simulink model "RequirementTable_testing_RA"  (R2022b)
settings: Solver=FixedStepAuto  StartTime=0.0  StopTime=10.0  FixedStep=1e-3  RelTol=1e-3  EnableMultiTasking=on
undefined symbols (not defined in the file): D0, D1, D10, D11, D12, D13, D2, D3, D4, D5, D6, D7, D8, D9, PTA0, PTA1, PTA2, PTB23, PTB9, PTC16, PTC17, PTC2, PTC3, PTC4, PTD0, PTD1, PTD2, PTD3
libraries: frdmk64flib x18, dspstat3 x1
settings Model: SimulationMode=external  ExtModeTrigDuration=5  Creator=sarahalabdulrazzak  LastModifiedBy=TheCoaler
settings SolverCC: AlgebraicLoopSolver=TrustRegion
settings OptimizationCC: EnhancedBackFolding=on  PassReuseOutputArgsAs=Individual arguments  ZeroExternalMemoryAtStartup=off  ZeroInternalMemoryAtStartup=off  MaxStackSize=64  OptimizeBlockOrder=speed  DifferentSizesBufferReuse=on  OptimizationCustomize=off  EfficientTunableParamExpr=on
settings DebuggingCC: ParameterTunabilityLossMsg=error  UnconnectedInputMsg=warning  UnconnectedOutputMsg=warning  UnconnectedLineMsg=warning  SFMachineParentedDataDiag=warning
settings HardwareCC: ProdBitPerPointer=32  ProdBitPerSizeT=32  ProdBitPerPtrDiffT=32  ProdLargestAtomicInteger=Long  ProdLargestAtomicFloat=Double  ProdWordSize=32  ProdHWDeviceType=ARM Compatible->ARM Cortex
settings ModelReferenceCC: EnableRefExpFcnMdlSchedulingChecks=on
settings SFSimCC: MATLABDynamicMemAlloc=off
settings RTWCC: Description=Embedded Coder  SystemTargetFile=ert.tlc  HardwareBoard=NXP FRDM-K64F  TLCOptions="-aInlineSetEventsForThisBaseRateFcn=TLC_FALSE -aSuppressMultiTaskScheduler=TLC_FALSE  -aRateBasedStepFcn=0"  TemplateMakefile=ert_default_tmf  Toolchain=GNU Tools for ARM Embedded Processors
settings CodeAppCC: ForceParamTrailComments=on  IgnoreCustomStorageClasses=off  OperatorAnnotations=on  SimulinkDataObjDesc=on  SFDataObjDesc=on  InsertBlockDesc=on
settings ERTTargetCC: ExtMode=on  ExtModeTransport=4  ExtModeMexFile=sendToCommService  ExtModeMexArgs='RA_Modes' 0

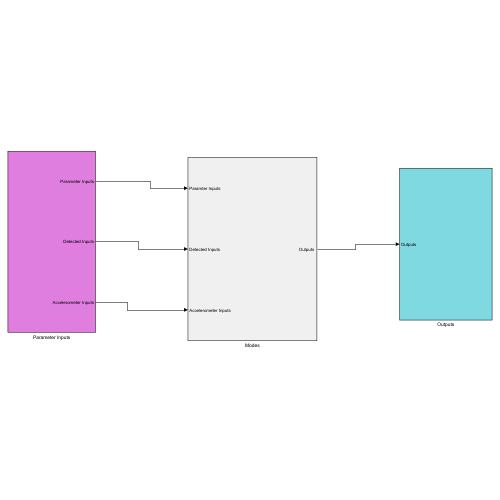
[thumbnail: Simulink's stored preview of the top-level diagram]
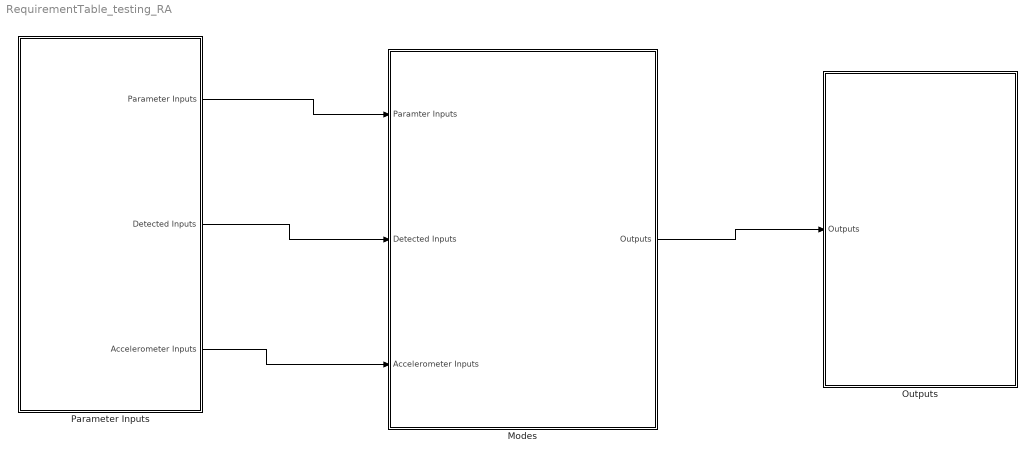
== system RequirementTable_testing_RA ==
  Modes : Subsystem
  Outputs : Subsystem
  Parameter Inputs : Subsystem
  wires:
  Parameter Inputs/1(Parameter Inputs) -> Modes/1(Paramter Inputs)
  Parameter Inputs/2(Detected Inputs) -> Modes/2(Detected Inputs)
  Modes/1("Outputs ") -> Outputs/1("Outputs ")
  Parameter Inputs/3(Accelerometer Inputs) -> Modes/3(Accelerometer Inputs)

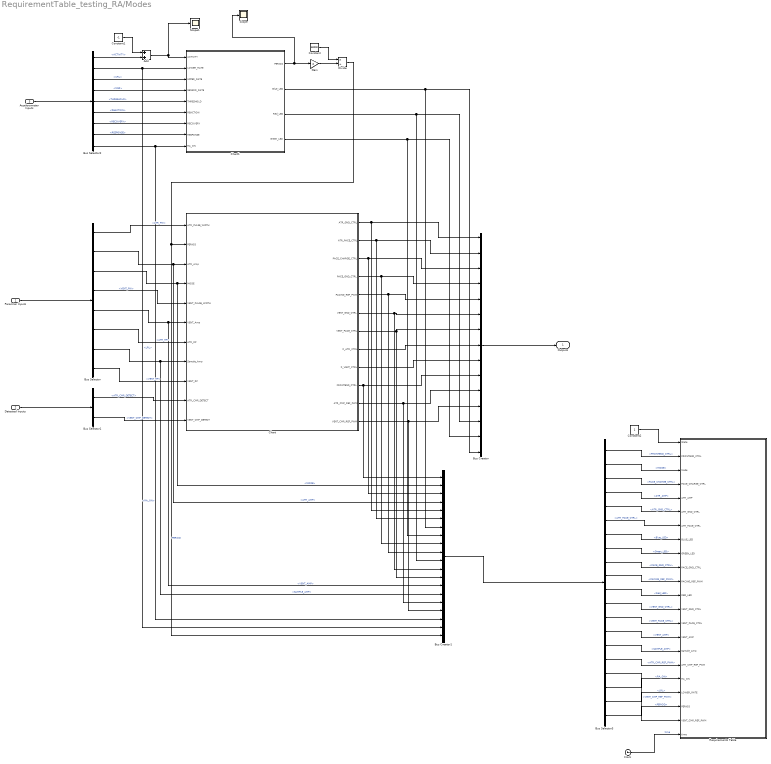
== system RequirementTable_testing_RA/Modes ==
  Paramter Inputs : Inport
  Detected Inputs : Inport  Port=2
  Accelerometer Inputs : Inport  Port=3
  Add : Sum
  Bus Creator : BusCreator  Inputs=15
  Bus Creator1 : BusCreator  Inputs=20
  Bus Selector : BusSelector  OutputSignals=ATR_PW,ATR_AMP,MODE,VENT_PW,VENT_AMP,ATR_RP,SAMPLE_AMP,VENT_RP
  Bus Selector1 : BusSelector  OutputSignals=ATR_CMP_DETECT,VENT_CMP_DETECT
  Bus Selector2 : BusSelector  OutputSignals=ACTIVITY,LRL,URL,MSR,THRESHOLD,REACTION,RECOVERY,RESPONSE,RA_ON
  Bus Selector3 : BusSelector  OutputSignals=FRONTEND_CTRL,MODE,PACE_CHARGE_CTRL,ATR_AMP,ATR_GND_CTRL,ATR_PACE_CTRL,Blue_LED,Green_LED,PACE_GND_CTRL,PACING_REF_PWM,Red_LED,VENT_GND_CTRL,VENT_PACE_CTRL,VENT_AMP,SAMPLE_AMP,ATR_CMP_REF_PWM,VENT_CMP_REF_PWM,RA_ON,LRL,PERIOD
  Chart : Stateflow chart  TreatAsAtomicUnit=on
  Chart1 : Stateflow chart  TreatAsAtomicUnit=on
  Clock : Clock
  Constant : Constant  Value=60000
  Constant1 : Constant  Value=-1
  Constant2 : Constant
  Divide : Product  Inputs=*/
  Gain : Gain  Gain=2
  Requirements Table : Requirements Table  TreatAsAtomicUnit=on
  Scope : Scope
  Scope1 : Scope
  "Outputs " : Outport
  wires:
  Paramter Inputs/1 -> Bus Selector/1
  Detected Inputs/1 -> Bus Selector1/1
  Bus Selector/1 -> Chart/1(ATR_PULSE_WIDTH)  "<ATR_PW>"
  Chart/1(ATR_GND_CTRL) -> Bus Creator1/5, Bus Creator/1
  Chart/2(ATR_PACE_CTRL) -> Bus Creator1/6, Bus Creator/2
  Chart/4(PACE_GND_CTRL) -> Bus Creator1/9, Bus Creator/4
  Chart/5(PACING_REF_PWM) -> Bus Creator1/10, Bus Creator/5
  Chart/6(VENT_GND_CTRL) -> Bus Creator1/12, Bus Creator/6
  Chart/7(VENT_PACE_CTRL) -> Bus Creator1/13, Bus Creator/7
  Chart/8(Z_ATR_CTRL) -> Bus Creator/8
  Chart/9(Z_VENT_CTRL) -> Bus Creator/9
  Chart/10(FRONTEND_CTRL) -> Bus Creator1/1, Bus Creator/10
  Chart/11(ATR_CMP_REF_PWM) -> Bus Creator1/16, Bus Creator/11
  Chart/12(VENT_CMP_REF_PWM) -> Bus Creator1/17, Bus Creator/12
  Bus Creator/1 -> "Outputs "/1
  Bus Selector1/1 -> Chart/10(ATR_CMP_DETECT)  "<ATR_CMP_DETECT>"
  Bus Selector1/2 -> Chart/11(VENT_CMP_DETECT)  "<VENT_CMP_DETECT>"
  Chart/3(PACE_CHARGE_CTRL) -> Bus Creator1/3, Bus Creator/3
  Bus Selector/2 -> Bus Creator1/4, Chart/3(ATR_Amp)  "<ATR_AMP>"
  Bus Selector/3 -> Bus Creator1/2, Chart/4(MODE)  "<MODE>"
  Bus Selector/4 -> Chart/5(VENT_PULSE_WIDTH)  "<VENT_PW>"
  Bus Selector/5 -> Bus Creator1/14, Chart/6(VENT_Amp)  "<VENT_AMP>"
  Bus Selector/6 -> Chart/7(ATR_RP)  "<ATR_RP>"
  Bus Selector/7 -> Bus Creator1/15, Chart/8(Sample_Amp)  "<SAMPLE_AMP>"
  Bus Selector/8 -> Chart/9(VENT_RP)  "<VENT_RP>"
  Accelerometer Inputs/1 -> Bus Selector2/1
  Bus Selector2/2 -> Bus Creator1/19, Chart1/2(LOWER_RATE)  "<LRL>"
  Bus Selector2/3 -> Chart1/3(UPPER_RATE)  "<URL>"
  Bus Selector2/4 -> Chart1/4(SENSOR_RATE)  "<MSR>"
  Bus Selector2/7 -> Chart1/7(RECOVERY)  "<RECOVERY>"
  Bus Selector2/8 -> Chart1/8(RESPONSE)  "<RESPONSE>"
  Bus Selector2/9 -> Bus Creator1/18, Chart1/9(RA_ON)  "<RA_ON>"
  Chart1/1(PERIOD) -> Scope/1, Gain/1
  Chart1/2(Blue_LED) -> Bus Creator1/7, Bus Creator/15
  Chart1/3(Red_LED) -> Bus Creator1/11, Bus Creator/13
  Chart1/4(Green_LED) -> Bus Creator1/8, Bus Creator/14
  Constant/1 -> Divide/1
  Divide/1 -> Bus Creator1/20, Chart/2(PERIOD)  "PERIOD"
  Gain/1 -> Divide/2
  Bus Selector2/5 -> Chart1/5(THRESHOLD)  "<THRESHOLD>"
  Bus Selector2/6 -> Chart1/6(REACTION)  "<REACTION>"
  Bus Selector2/1 -> Add/2  "<ACTIVITY>"
  Add/1 -> Scope1/1, Chart1/1(ACTIVITY)
  Constant1/1 -> Add/1
  Bus Creator1/1 -> Bus Selector3/1
  Bus Selector3/1 -> Requirements Table/2(FRONTEND_CTRL)  "<FRONTEND_CTRL>"
  Bus Selector3/2 -> Requirements Table/3(Mode)  "<MODE>"
  Bus Selector3/3 -> Requirements Table/4(PACE_CHARGE_CTRL)  "<PACE_CHARGE_CTRL>"
  Bus Selector3/4 -> Requirements Table/5(ATR_AMP)  "<ATR_AMP>"
  Bus Selector3/5 -> Requirements Table/6(ATR_GND_CTRL)  "<ATR_GND_CTRL>"
  Bus Selector3/6 -> Requirements Table/7(ATR_PACE_CTRL)  "<ATR_PACE_CTRL>"
  Bus Selector3/7 -> Requirements Table/8(BLUE_LED)  "<Blue_LED>"
  Bus Selector3/8 -> Requirements Table/9(GREEN_LED)  "<Green_LED>"
  Bus Selector3/9 -> Requirements Table/10(PACE_GND_CTRL)  "<PACE_GND_CTRL>"
  Bus Selector3/10 -> Requirements Table/11(PACING_REF_PWM)  "<PACING_REF_PWM>"
  Bus Selector3/11 -> Requirements Table/12(RED_LED)  "<Red_LED>"
  Bus Selector3/12 -> Requirements Table/13(VENT_GND_CTRL)  "<VENT_GND_CTRL>"
  Bus Selector3/13 -> Requirements Table/14(VENT_PACE_CTRL)  "<VENT_PACE_CTRL>"
  Bus Selector3/14 -> Requirements Table/15(VENT_AMP)  "<VENT_AMP>"
  Bus Selector3/15 -> Requirements Table/16(Sample_Amp)  "<SAMPLE_AMP>"
  Bus Selector3/16 -> Requirements Table/17(ATR_CMP_REF_PWM)  "<ATR_CMP_REF_PWM>"
  Bus Selector3/19 -> Requirements Table/19(LOWER_RATE)  "<LRL>"
  Constant2/1 -> Requirements Table/1(State)
  Bus Selector3/20 -> Requirements Table/20(PERIOD)  "<PERIOD>"
  Bus Selector3/18 -> Requirements Table/18(RA_ON)  "<RA_ON>"
  Bus Selector3/17 -> Requirements Table/21(VENT_CMP_REF_PWM)  "<VENT_CMP_REF_PWM>"
  Clock/1 -> Requirements Table/22(time)  "time"

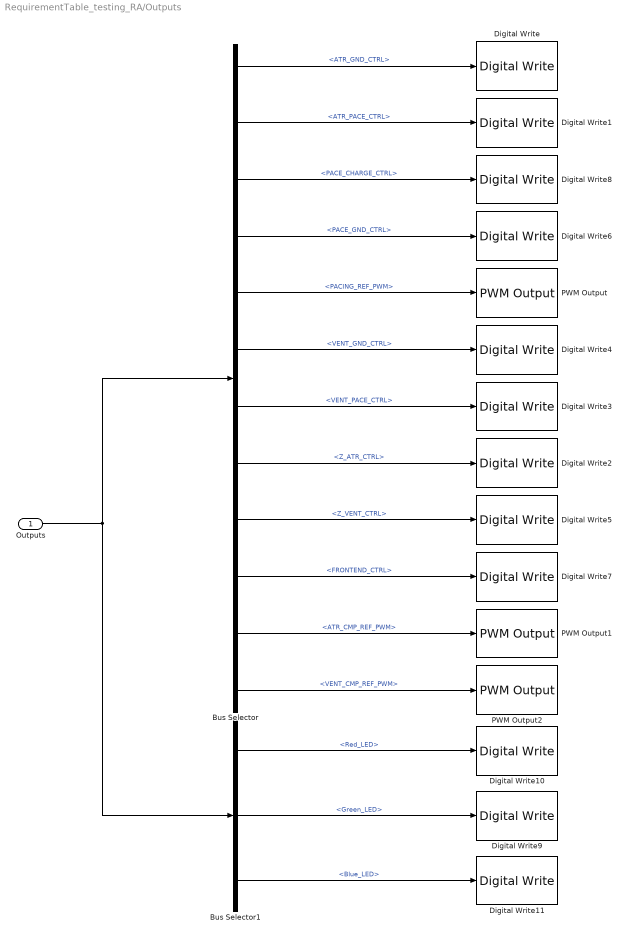
== system RequirementTable_testing_RA/Outputs ==
  "Outputs " : Inport
  Bus Selector : BusSelector  OutputSignals=ATR_GND_CTRL,ATR_PACE_CTRL,PACE_CHARGE_CTRL,PACE_GND_CTRL,PACING_REF_PWM,VENT_GND_CTRL,VENT_PACE_CTRL,Z_ATR_CTRL,Z_VENT_CTRL,FRONTEND_CTRL,ATR_CMP_REF_PWM,VENT_CMP_REF_PWM
  Bus Selector1 : BusSelector  OutputSignals=Red_LED,Green_LED,Blue_LED
  Digital Write : frdmk64flib/Digital Write  Whichpin=PTD2 (D11)
  Digital Write1 : frdmk64flib/Digital Write  Whichpin=PTA0 (D8)
  Digital Write10 : frdmk64flib/Digital Write  Whichpin=RED_LED
  Digital Write11 : frdmk64flib/Digital Write  Whichpin=BLUE_LED
  Digital Write2 : frdmk64flib/Digital Write  Whichpin=PTB23 (D4)
  Digital Write3 : frdmk64flib/Digital Write  Whichpin=PTC4 (D9)
  Digital Write4 : frdmk64flib/Digital Write  Whichpin=PTD3 (D12)
  Digital Write5 : frdmk64flib/Digital Write  Whichpin=PTC3 (D7)
  Digital Write6 : frdmk64flib/Digital Write  Whichpin=PTD0 (D10)
  Digital Write7 : frdmk64flib/Digital Write  Whichpin=PTD1 (D13)
  Digital Write8 : frdmk64flib/Digital Write  Whichpin=PTB9 (D2)
  Digital Write9 : frdmk64flib/Digital Write  Whichpin=GREEN_LED
  PWM Output : frdmk64flib/PWM Output  Whichpin=PTA2 (D5)  InitialFrequency=2000  InitialDutyCycle=0
  PWM Output1 : frdmk64flib/PWM Output  Whichpin=PTC2 (D6)  InitialFrequency=2000  InitialDutyCycle=0
  PWM Output2 : frdmk64flib/PWM Output  Whichpin=PTA1 (D3)  InitialFrequency=2000  InitialDutyCycle=0
  wires:
  Bus Selector/1 -> Digital Write/1  "<ATR_GND_CTRL>"
  Bus Selector/2 -> Digital Write1/1  "<ATR_PACE_CTRL>"
  Bus Selector/3 -> Digital Write8/1  "<PACE_CHARGE_CTRL>"
  Bus Selector/4 -> Digital Write6/1  "<PACE_GND_CTRL>"
  Bus Selector/5 -> PWM Output/1  "<PACING_REF_PWM>"
  Bus Selector/6 -> Digital Write4/1  "<VENT_GND_CTRL>"
  Bus Selector/7 -> Digital Write3/1  "<VENT_PACE_CTRL>"
  Bus Selector/8 -> Digital Write2/1  "<Z_ATR_CTRL>"
  Bus Selector/9 -> Digital Write5/1  "<Z_VENT_CTRL>"
  Bus Selector/10 -> Digital Write7/1  "<FRONTEND_CTRL>"
  Bus Selector/11 -> PWM Output1/1  "<ATR_CMP_REF_PWM>"
  Bus Selector/12 -> PWM Output2/1  "<VENT_CMP_REF_PWM>"
  "Outputs "/1 -> Bus Selector/1, Bus Selector1/1
  Bus Selector1/1 -> Digital Write10/1  "<Red_LED>"
  Bus Selector1/2 -> Digital Write9/1  "<Green_LED>"
  Bus Selector1/3 -> Digital Write11/1  "<Blue_LED>"

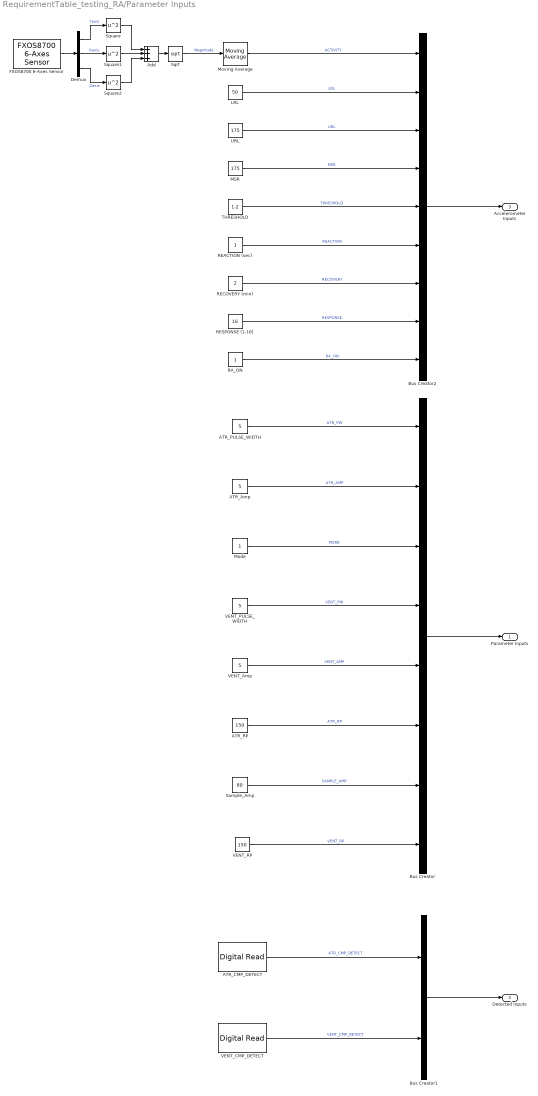
== system RequirementTable_testing_RA/Parameter Inputs ==
  ATR_Amp : Constant  Value=5
  ATR_CMP_DETECT : frdmk64flib/Digital Read  Whichpin=PTC16 (D0)  SampleTime=-1
  ATR_PULSE_WIDTH : Constant  Value=5
  ATR_RP : Constant  Value=150
  Add : Sum  Inputs=+++
  Bus Creator : BusCreator  Inputs=8
  Bus Creator1 : BusCreator  Inputs=2
  Bus Creator2 : BusCreator  Inputs=9
  Demux : Demux  Outputs=3
  FXOS8700 6-Axes Sensor : frdmk64flib/FXOS8700 6-Axes Sensor  Activesensor=Accelerometer only  ODR=800Hz  HybridODR=400Hz  Accelfullrange=-4g to +4g  SampleTime=-1
  LRL : Constant  Value=50  OutDataTypeStr=double
  MSR : Constant  Value=175  OutDataTypeStr=double
  Mode : Constant
  Moving Average : dspstat3/Moving Average  Method=Exponential weighting  ForgettingFactorPort=off  SpecifyWindowLength=on  WindowLength=4  OverlapLength=3  AllowArbitraryInputLength=off  ForgettingFactor=0.999  SimulateUsing=Code generation
  RA_ON : Constant  OutDataTypeStr=boolean
  REACTION (sec) : Constant  OutDataTypeStr=double
  RECOVERY (min) : Constant  Value=2  OutDataTypeStr=double
  RESPONSE (1-16) : Constant  Value=16  OutDataTypeStr=double
  Sample_Amp : Constant  Value=80
  Sqrt : Sqrt
  Square : Math  Operator=square
  Square1 : Math  Operator=square
  Square2 : Math  Operator=square
  THRESHOLD : Constant  Value=1.2  OutDataTypeStr=double
  URL : Constant  Value=175  OutDataTypeStr=double
  VENT_Amp : Constant  Value=5
  VENT_CMP_DETECT : frdmk64flib/Digital Read  Whichpin=PTC17 (D1)  SampleTime=-1
  VENT_PULSE_WIDTH : Constant  Value=5
  VENT_RP : Constant  Value=150
  Parameter Inputs : Outport
  Detected Inputs : Outport  Port=2
  Accelerometer Inputs : Outport  Port=3
  wires:
  Bus Creator/1 -> Parameter Inputs/1
  ATR_PULSE_WIDTH/1 -> Bus Creator/1  "ATR_PW"
  ATR_Amp/1 -> Bus Creator/2  "ATR_AMP"
  Mode/1 -> Bus Creator/3  "MODE"
  VENT_PULSE_WIDTH/1 -> Bus Creator/4  "VENT_PW"
  VENT_Amp/1 -> Bus Creator/5  "VENT_AMP"
  ATR_RP/1 -> Bus Creator/6  "ATR_RP"
  Sample_Amp/1 -> Bus Creator/7  "SAMPLE_AMP"
  VENT_RP/1 -> Bus Creator/8  "VENT_RP"
  Bus Creator1/1 -> Detected Inputs/1
  VENT_CMP_DETECT/1 -> Bus Creator1/2  "VENT_CMP_DETECT"
  ATR_CMP_DETECT/1 -> Bus Creator1/1  "ATR_CMP_DETECT"
  Sqrt/1 -> Moving Average/1  "Magnitude"
  Demux/3 -> Square2/1  "Zaxis"
  Square2/1 -> Add/3
  Add/1 -> Sqrt/1
  Demux/2 -> Square1/1  "Xaxis"
  Square/1 -> Add/1
  Demux/1 -> Square/1  "Yaxis"
  FXOS8700 6-Axes Sensor/1 -> Demux/1
  Square1/1 -> Add/2
  Bus Creator2/1 -> Accelerometer Inputs/1
  Moving Average/1 -> Bus Creator2/1  "ACTIVITY"
  LRL/1 -> Bus Creator2/2  "LRL"
  URL/1 -> Bus Creator2/3  "URL"
  MSR/1 -> Bus Creator2/4  "MSR"
  RA_ON/1 -> Bus Creator2/9  "RA_ON"
  REACTION (sec)/1 -> Bus Creator2/6  "REACTION"
  THRESHOLD/1 -> Bus Creator2/5  "THRESHOLD"
  RECOVERY (min)/1 -> Bus Creator2/7  "RECOVERY"
  RESPONSE (1-16)/1 -> Bus Creator2/8  "RESPONSE"

== stateflow chart RequirementTable_testing_RA/Modes/Chart1 ==
  state RECOVER_RATE
    %this is for if the RA is turned off while the
    %slowly shift activity (might not need)
    %if the period is above LRL, reduce by amount that will bring diff to 0 within recovery time
    Green_LED = true
    AVG_ACT = ACTIVITY
    if PERIOD > LOWER_RATE
    PERIOD = PERIOD - (SENSOR_RATE-LOWER_RATE)/(RECOVERY*1000)
    DELAY = (RECOVERY*1000)
    else
    PERIOD = LOWER_RATE
    DELAY = 0
    end
  state RA_OFF
    %set the period to LRL
    %read current activity
    %and assign to var.
    entry:
    PERIOD = LOWER_RATE
    AVG_ACT = ACTIVITY
    TH = single(THRESHOLD)
  state SET_TARGET
    %set the target rate and make sure it falls within the bounds
    Green_LED = false
    Red_LED = true
    TARGET_RATE = RESPONSE*((SENSOR_RATE - LOWER_RATE)/10)*ACTIVITY + LOWER_RATE
    %TARGET_RATE = 120
    if TARGET_RATE > SENSOR_RATE
    TARGET_RATE = SENSOR_RATE
    elseif TARGET_RATE < LOWER_RATE
    TARGET_RATE = LOWER_RATE
    end
  state RA_ON
    entry:
    Blue_LED = false
    Green_LED = false
    %Red_LED = false
  state RECOVER_REACT
    %slowly shift activity (might not need)
    %if Period is above target, decrease using recovery
    %if below target, increase using reaction
    Blue_LED = true
    AVG_ACT = ACTIVITY
    if PERIOD > TARGET_RATE
    PERIOD = PERIOD - (SENSOR_RATE-LOWER_RATE)/(RECOVERY*1000)
    DELAY = (RECOVERY*1000)
    elseif PERIOD < TARGET_RATE
    PERIOD = PERIOD + (SENSOR_RATE-LOWER_RATE)/(REACTION*1000)
    DELAY = (REACTION*1000)
    end
  RECOVER_RATE -> SET_TARGET [order 1] : [n >= DELAY && AVG_ACT >= TH]
  RECOVER_RATE -> RECOVER_RATE [order 2] : after(1,msec){n = n+1}
  RECOVER_RATE -> RA_OFF [order 3] : [RA_ON == FALSE && n >= DELAY]
  RA_ON -> RECOVER_RATE [order 1] : [AVG_ACT < TH]{n=0}
  (default) -> RA_OFF
  RA_ON -> SET_TARGET [order 2] : [AVG_ACT >= TH]
  RA_OFF -> RA_ON : [RA_ON == TRUE]{TARGET_RATE=PERIOD}
  RECOVER_REACT -> RA_ON [order 1] : [n >= DELAY]
  SET_TARGET -> RECOVER_REACT : {n=0, AVG_ACT = ACTIVITY}
  RECOVER_REACT -> RECOVER_REACT [order 2] : after(1,msec){n = n+1}
  data: ACTIVITY input; LOWER_RATE input; UPPER_RATE input; SENSOR_RATE input; THRESHOLD input; REACTION input; RECOVERY input; RESPONSE input; RA_ON input; PERIOD output double; TRUE local =1; FALSE local =0; TARGET_RATE local double; DELAY local double; n local; Blue_LED output; Red_LED output; Green_LED output; TH local; AVG_ACT local

== stateflow chart RequirementTable_testing_RA/Modes/Requirements Table ==
  (default) -> (junction 1073748085)
  (junction 1073748085) -> (junction 1073748086) : {
      | % SF_REQ_REV_07
      | }
  (junction 1073748086) -> (junction 1073748088) : {
      | % HEADER_ASSIGNMENTS
      |
      | }
  (junction 1073748088) -> (junction 1073748418) : {
      | % START_A_28
      | }
  (junction 1073748418) -> (junction 1073748420) : {
      | }
  (junction 1073748420) -> (junction 1073748422) : {
      | reqtable_assumption((Mode<=4), 28);
      | }
  (junction 1073748422) -> (junction 1073748424) : {
      | }
  (junction 1073748424) -> (junction 1073748426) : {
      | % START_A_109
      | }
  (junction 1073748426) -> (junction 1073748428) : {
      | }
  (junction 1073748428) -> (junction 1073748430) : {
      | reqtable_assumption((Mode>=1), 109);
      | }
  (junction 1073748430) -> (junction 1073748432) : {
      | }
  (junction 1073748432) -> (junction 1073748434) : {
      | % END_A_109
      | }
  (junction 1073748434) -> (junction 1073748440) : {
      | % START_A_112
      | }
  (junction 1073748440) -> (junction 1073748442) : {
      | }
  (junction 1073748442) -> (junction 1073748444) : {
      | reqtable_assumption((rem(Mode,1)<=0), 112);
      | }
  (junction 1073748444) -> (junction 1073748446) : {
      | }
  (junction 1073748446) -> (junction 1073748448) : {
      | % END_A_112
      | }
  (junction 1073748448) -> (junction 1073748436) : {
      | % END_A_28
      | }
  (junction 1073748436) -> (junction 1073748464) : {
      | % START_A_106
      | }
  (junction 1073748464) -> (junction 1073748466) : {
      | }
  (junction 1073748466) -> (junction 1073748468) : {
      | reqtable_assumption((State<=1), 106);
      | }
  (junction 1073748468) -> (junction 1073748470) : {
      | }
  (junction 1073748470) -> (junction 1073748472) : {
      | % START_A_118
      | }
  (junction 1073748472) -> (junction 1073748474) : {
      | }
  (junction 1073748474) -> (junction 1073748476) : {
      | reqtable_assumption((State>=0), 118);
      | }
  (junction 1073748476) -> (junction 1073748478) : {
      | }
  (junction 1073748478) -> (junction 1073748480) : {
      | % END_A_118
      | }
  (junction 1073748480) -> (junction 1073748482) : {
      | % END_A_106
      | }
  (junction 1073748482) -> (junction 1073748486) : {
      | % START_A_115
      | }
  (junction 1073748486) -> (junction 1073748488) : {
      | }
  (junction 1073748488) -> (junction 1073748490) : {
      | reqtable_assumption((FRONTEND_CTRL<=1), 115);
      | }
  (junction 1073748490) -> (junction 1073748492) : {
      | }
  (junction 1073748492) -> (junction 1073748494) : {
      | % START_A_121
      | }
  (junction 1073748494) -> (junction 1073748496) : {
      | }
  (junction 1073748496) -> (junction 1073748498) : {
      | reqtable_assumption((FRONTEND_CTRL>=0), 121);
      | }
  (junction 1073748498) -> (junction 1073748500) : {
      | }
  (junction 1073748500) -> (junction 1073748502) : {
      | % END_A_121
      | }
  (junction 1073748502) -> (junction 1073748504) : {
      | % END_A_115
      | }
  (junction 1073748504) -> (junction 1073748100) : {
      | % START_R_1
      | }
  (junction 1073748100) -> (junction 1073748102) : {
      | }
  (junction 1073748102) -> (junction 1073748104)
  (junction 1073748104) -> (junction 1073748106) [order 1] : [(((RA_ON) == (0))) && (((Mode) == (1))) && (((State) == (0)))]
  (junction 1073748104) -> (junction 1073748112) [order 2]
  (junction 1073748106) -> (junction 1073748108) : {
      | reqtable_postcondition((((PACE_CHARGE_CTRL) == (1))) && (ATR_PACE_CTRL == 0) && (((PACING_REF_PWM ) == (ATR_AMP))) && (((PACE_CHARGE_CTRL) == (1))) && (((PACE_GND_CTRL) == (1))) && (ATR_GND_CTRL == 1) && (((RED_LED) == (0))) && (((GREEN_LED) == (0))) && (((BLUE_LED) == (0))) && (time-oldTime / (60*1000) >= LOWER_RATE), 'R:1');
      |
      | }
  (junction 1073748108) -> (junction 1073748110) : {
      | }
  (junction 1073748110) -> (junction 1073748112)
  (junction 1073748112) -> (junction 1073748114)
  (junction 1073748114) -> (junction 1073748116) : {
      | % END_R_1
      | }
  (junction 1073748116) -> (junction 1073748118) : {
      | % START_R_82
      | }
  (junction 1073748118) -> (junction 1073748120) : {
      | }
  (junction 1073748120) -> (junction 1073748122)
  (junction 1073748122) -> (junction 1073748124) [order 1] : [(((RA_ON) == (1))) && (((Mode) == (1))) && (((State) == (0)))]
  (junction 1073748122) -> (junction 1073748130) [order 2]
  (junction 1073748124) -> (junction 1073748126) : {
      | reqtable_postcondition((((PACE_CHARGE_CTRL) == (1))) && (ATR_PACE_CTRL == 0) && (((PACING_REF_PWM ) == (ATR_AMP))) && (((PACE_CHARGE_CTRL) == (1))) && (((PACE_GND_CTRL) == (1))) && (ATR_GND_CTRL == 1) && (((RED_LED) == (0))) && (((GREEN_LED) == (0))) && (((BLUE_LED) == (0))) && (time-oldTime >= PERIOD-5), 'R:2');
      |
      | }
  (junction 1073748126) -> (junction 1073748128) : {
      | }
  (junction 1073748128) -> (junction 1073748130)
  (junction 1073748130) -> (junction 1073748132)
  (junction 1073748132) -> (junction 1073748134) : {
      | % END_R_82
      | }
  (junction 1073748134) -> (junction 1073748136) : {
      | % START_R_7
      | }
  (junction 1073748136) -> (junction 1073748138) : {
      | }
  (junction 1073748138) -> (junction 1073748140)
  (junction 1073748140) -> (junction 1073748142) [order 1] : [(((RA_ON) == (0))) && (((Mode) == (1))) && (((State) == (1)))]
  (junction 1073748140) -> (junction 1073748148) [order 2]
  (junction 1073748142) -> (junction 1073748144) : {
      | reqtable_postcondition((((PACE_CHARGE_CTRL) == (0))) && (ATR_PACE_CTRL == 1) && (((PACING_REF_PWM ) == (ATR_AMP))) && (((PACE_CHARGE_CTRL) == (0))) && (((PACE_GND_CTRL) == (1))) && (ATR_GND_CTRL == 0) && (((RED_LED) == (1))) && (((GREEN_LED) == (0))) && (((BLUE_LED) == (0))) && (time-oldTime / (60*1000) >= LOWER_RATE), 'R:3');
      |
      | }
  (junction 1073748144) -> (junction 1073748146) : {
      | }
  (junction 1073748146) -> (junction 1073748148)
  (junction 1073748148) -> (junction 1073748150)
  (junction 1073748150) -> (junction 1073748152) : {
      | % END_R_7
      | }
  (junction 1073748152) -> (junction 1073748154) : {
      | % START_R_88
      | }
  (junction 1073748154) -> (junction 1073748156) : {
      | }
  (junction 1073748156) -> (junction 1073748158)
  (junction 1073748158) -> (junction 1073748160) [order 1] : [(((RA_ON) == (1))) && (((Mode) == (1))) && (((State) == (1)))]
  (junction 1073748158) -> (junction 1073748166) [order 2]
  (junction 1073748160) -> (junction 1073748162) : {
      | reqtable_postcondition((((PACE_CHARGE_CTRL) == (0))) && (ATR_PACE_CTRL == 1) && (((PACING_REF_PWM ) == (ATR_AMP))) && (((PACE_CHARGE_CTRL) == (0))) && (((PACE_GND_CTRL) == (1))) && (ATR_GND_CTRL == 0) && (((RED_LED) == (1))) && (((GREEN_LED) == (0))) && (((BLUE_LED) == (0))) && (time-oldTime >= PERIOD-5), 'R:4');
      |
      | }
  (junction 1073748162) -> (junction 1073748164) : {
      | }
  (junction 1073748164) -> (junction 1073748166)
  (junction 1073748166) -> (junction 1073748168)
  (junction 1073748168) -> (junction 1073748170) : {
      | % END_R_88
      | }
  (junction 1073748170) -> (junction 1073748172) : {
      | % START_R_10
      | }
  (junction 1073748172) -> (junction 1073748174) : {
      | }
  (junction 1073748174) -> (junction 1073748176)
  (junction 1073748176) -> (junction 1073748178) [order 1] : [(((RA_ON) == (0))) && (((Mode) == (3))) && (((State) == (0)))]
  (junction 1073748176) -> (junction 1073748184) [order 2]
  (junction 1073748178) -> (junction 1073748180) : {
      | reqtable_postcondition((((PACE_CHARGE_CTRL) == (1))) && (VENT_PACE_CTRL == 0) && (((PACING_REF_PWM ) == (VENT_AMP))) && (((PACE_CHARGE_CTRL) == (1))) && (((PACE_GND_CTRL) == (1))) && (VENT_GND_CTRL == 1) && (((RED_LED) == (0))) && (((GREEN_LED) == (0))) && (((BLUE_LED) == (0))) && (time-oldTime / (60*1000) >= LOWER_RATE), 'R:5');
      |
      | }
  (junction 1073748180) -> (junction 1073748182) : {
      | }
  (junction 1073748182) -> (junction 1073748184)
  (junction 1073748184) -> (junction 1073748186)
  (junction 1073748186) -> (junction 1073748188) : {
      | % END_R_10
      | }
  (junction 1073748188) -> (junction 1073748190) : {
      | % START_R_85
      | }
  (junction 1073748190) -> (junction 1073748192) : {
      | }
  (junction 1073748192) -> (junction 1073748194)
  (junction 1073748194) -> (junction 1073748196) [order 1] : [(((RA_ON) == (1))) && (((Mode) == (3))) && (((State) == (0)))]
  (junction 1073748194) -> (junction 1073748202) [order 2]
  (junction 1073748196) -> (junction 1073748198) : {
      | reqtable_postcondition((((PACE_CHARGE_CTRL) == (1))) && (VENT_PACE_CTRL == 0) && (((PACING_REF_PWM ) == (VENT_AMP))) && (((PACE_CHARGE_CTRL) == (1))) && (((PACE_GND_CTRL) == (1))) && (VENT_GND_CTRL == 1) && (((RED_LED) == (0))) && (((GREEN_LED) == (0))) && (((BLUE_LED) == (0))) && (time-oldTime >= PERIOD-5), 'R:6');
      |
      | }
  (junction 1073748198) -> (junction 1073748200) : {
      | }
  (junction 1073748200) -> (junction 1073748202)
  (junction 1073748202) -> (junction 1073748204)
  (junction 1073748204) -> (junction 1073748206) : {
      | % END_R_85
      | }
  (junction 1073748206) -> (junction 1073748208) : {
      | % START_R_13
      | }
  (junction 1073748208) -> (junction 1073748210) : {
      | }
  (junction 1073748210) -> (junction 1073748212)
  (junction 1073748212) -> (junction 1073748214) [order 1] : [(((RA_ON) == (0))) && (((Mode) == (3))) && (((State) == (1)))]
  (junction 1073748212) -> (junction 1073748220) [order 2]
  (junction 1073748214) -> (junction 1073748216) : {
      | reqtable_postcondition((((PACE_CHARGE_CTRL) == (0))) && (VENT_PACE_CTRL == 1) && (((PACING_REF_PWM ) == (VENT_AMP))) && (((PACE_CHARGE_CTRL) == (0))) && (((PACE_GND_CTRL) == (1))) && (VENT_GND_CTRL == 0) && (((RED_LED) == (0))) && (((GREEN_LED) == (1))) && (((BLUE_LED) == (0))) && (time-oldTime / (60*1000) >= LOWER_RATE), 'R:7');
      |
      | }
  (junction 1073748216) -> (junction 1073748218) : {
      | }
  (junction 1073748218) -> (junction 1073748220)
  (junction 1073748220) -> (junction 1073748222)
  (junction 1073748222) -> (junction 1073748224) : {
      | % END_R_13
      | }
  (junction 1073748224) -> (junction 1073748226) : {
      | % START_R_91
      | }
  (junction 1073748226) -> (junction 1073748228) : {
      | }
  (junction 1073748228) -> (junction 1073748230)
  (junction 1073748230) -> (junction 1073748232) [order 1] : [(((RA_ON) == (1))) && (((Mode) == (3))) && (((State) == (1)))]
  (junction 1073748230) -> (junction 1073748238) [order 2]
  (junction 1073748232) -> (junction 1073748234) : {
      | reqtable_postcondition((((PACE_CHARGE_CTRL) == (0))) && (VENT_PACE_CTRL == 1) && (((PACING_REF_PWM ) == (VENT_AMP))) && (((PACE_CHARGE_CTRL) == (0))) && (((PACE_GND_CTRL) == (1))) && (VENT_GND_CTRL == 0) && (((RED_LED) == (0))) && (((GREEN_LED) == (1))) && (((BLUE_LED) == (0))) && (time-oldTime >= PERIOD-5), 'R:8');
      |
      | }
  (junction 1073748234) -> (junction 1073748236) : {
      | }
  (junction 1073748236) -> (junction 1073748238)
  (junction 1073748238) -> (junction 1073748240)
  (junction 1073748240) -> (junction 1073748242) : {
      | % END_R_91
      | }
  (junction 1073748242) -> (junction 1073748244) : {
      | % START_R_16
      | }
  (junction 1073748244) -> (junction 1073748246) : {
      | }
  (junction 1073748246) -> (junction 1073748248)
  (junction 1073748248) -> (junction 1073748250) [order 1] : [(((RA_ON) == (0))) && (((Mode) == (2))) && (((State) == (0))) && (FRONTEND_CTRL == 1)]
  (junction 1073748248) -> (junction 1073748256) [order 2]
  (junction 1073748250) -> (junction 1073748252) : {
      | reqtable_postcondition((((PACE_CHARGE_CTRL) == (1))) && (ATR_PACE_CTRL == 0) && (((PACING_REF_PWM ) == (ATR_AMP))) && (((PACE_CHARGE_CTRL) == (1))) && (((PACE_GND_CTRL) == (1))) && (ATR_GND_CTRL == 1) && (((RED_LED) == (0))) && (((GREEN_LED) == (0))) && (((BLUE_LED) == (0))) && (ATR_CMP_REF_PWM == Sample_Amp) && (time-oldTime / (60*1000) >= LOWER_RATE), 'R:9');
      |
      | }
  (junction 1073748252) -> (junction 1073748254) : {
      | }
  (junction 1073748254) -> (junction 1073748256)
  (junction 1073748256) -> (junction 1073748258)
  (junction 1073748258) -> (junction 1073748260) : {
      | % END_R_16
      | }
  (junction 1073748260) -> (junction 1073748262) : {
      | % START_R_94
      | }
  (junction 1073748262) -> (junction 1073748264) : {
      | }
  (junction 1073748264) -> (junction 1073748266)
  (junction 1073748266) -> (junction 1073748268) [order 1] : [(((RA_ON) == (1))) && (((Mode) == (2))) && (((State) == (0))) && (FRONTEND_CTRL == 1)]
  (junction 1073748266) -> (junction 1073748274) [order 2]
  (junction 1073748268) -> (junction 1073748270) : {
      | reqtable_postcondition((((PACE_CHARGE_CTRL) == (1))) && (ATR_PACE_CTRL == 0) && (((PACING_REF_PWM ) == (ATR_AMP))) && (((PACE_CHARGE_CTRL) == (1))) && (((PACE_GND_CTRL) == (1))) && (ATR_GND_CTRL == 1) && (((RED_LED) == (0))) && (((GREEN_LED) == (0))) && (((BLUE_LED) == (0))) && (ATR_CMP_REF_PWM == Sample_Amp) && (time-oldTime >= PERIOD-5), 'R:10');
      |
      | }
  (junction 1073748270) -> (junction 1073748272) : {
      | }
  (junction 1073748272) -> (junction 1073748274)
  (junction 1073748274) -> (junction 1073748276)
  (junction 1073748276) -> (junction 1073748278) : {
      | % END_R_94
      | }
  (junction 1073748278) -> (junction 1073748280) : {
      | % START_R_19
      | }
  (junction 1073748280) -> (junction 1073748282) : {
      | }
  (junction 1073748282) -> (junction 1073748284)
  (junction 1073748284) -> (junction 1073748286) [order 1] : [(((RA_ON) == (0))) && (((Mode) == (2))) && (((State) == (1)))]
  (junction 1073748284) -> (junction 1073748292) [order 2]
  (junction 1073748286) -> (junction 1073748288) : {
      | reqtable_postcondition((((PACE_CHARGE_CTRL) == (0))) && (ATR_PACE_CTRL == 1) && (((PACING_REF_PWM ) == (ATR_AMP))) && (((PACE_CHARGE_CTRL) == (0))) && (((PACE_GND_CTRL) == (1))) && (ATR_GND_CTRL == 0) && (((RED_LED) == (0))) && (((GREEN_LED) == (0))) && (((BLUE_LED) == (0))) && (ATR_CMP_REF_PWM == Sample_Amp) && (time-oldTime / (60*1000) >= LOWER_RATE), 'R:11');
      |
      | }
  (junction 1073748288) -> (junction 1073748290) : {
      | }
  (junction 1073748290) -> (junction 1073748292)
  (junction 1073748292) -> (junction 1073748294)
  (junction 1073748294) -> (junction 1073748296) : {
      | % END_R_19
      | }
  (junction 1073748296) -> (junction 1073748298) : {
      | % START_R_97
      | }
  (junction 1073748298) -> (junction 1073748300) : {
      | }
  (junction 1073748300) -> (junction 1073748302)
  (junction 1073748302) -> (junction 1073748304) [order 1] : [(((RA_ON) == (1))) && (((Mode) == (2))) && (((State) == (1)))]
  (junction 1073748302) -> (junction 1073748310) [order 2]
  (junction 1073748304) -> (junction 1073748306) : {
      | reqtable_postcondition((((PACE_CHARGE_CTRL) == (0))) && (ATR_PACE_CTRL == 1) && (((PACING_REF_PWM ) == (ATR_AMP))) && (((PACE_CHARGE_CTRL) == (0))) && (((PACE_GND_CTRL) == (1))) && (ATR_GND_CTRL == 0) && (((RED_LED) == (0))) && (((GREEN_LED) == (0))) && (((BLUE_LED) == (0))) && (ATR_CMP_REF_PWM == Sample_Amp) && (time-oldTime >= PERIOD-5), 'R:12');
      |
      | }
  (junction 1073748306) -> (junction 1073748308) : {
      | }
  (junction 1073748308) -> (junction 1073748310)
  (junction 1073748310) -> (junction 1073748312)
  (junction 1073748312) -> (junction 1073748314) : {
      | % END_R_97
      | }
  (junction 1073748314) -> (junction 1073748316) : {
      | % START_R_22
      | }
  (junction 1073748316) -> (junction 1073748318) : {
      | }
  (junction 1073748318) -> (junction 1073748320)
  (junction 1073748320) -> (junction 1073748322) [order 1] : [(((RA_ON) == (0))) && (((Mode) == (4))) && (((State) == (0))) && (FRONTEND_CTRL == 1)]
  (junction 1073748320) -> (junction 1073748328) [order 2]
  (junction 1073748322) -> (junction 1073748324) : {
      | reqtable_postcondition((((PACE_CHARGE_CTRL) == (1))) && (VENT_PACE_CTRL == 0) && (((PACING_REF_PWM ) == (VENT_AMP))) && (((PACE_CHARGE_CTRL) == (1))) && (((PACE_GND_CTRL) == (1))) && (VENT_GND_CTRL == 1) && (((RED_LED) == (0))) && (((GREEN_LED) == (0))) && (((BLUE_LED) == (0))) && (VENT_CMP_REF_PWM == Sample_Amp) && (time-oldTime / (60*1000) >= LOWER_RATE), 'R:13');
      |
      | }
  (junction 1073748324) -> (junction 1073748326) : {
      | }
  (junction 1073748326) -> (junction 1073748328)
  (junction 1073748328) -> (junction 1073748330)
  (junction 1073748330) -> (junction 1073748332) : {
      | % END_R_22
      | }
  (junction 1073748332) -> (junction 1073748334) : {
      | % START_R_100
      | }
  (junction 1073748334) -> (junction 1073748336) : {
      | }
  (junction 1073748336) -> (junction 1073748338)
  (junction 1073748338) -> (junction 1073748340) [order 1] : [(((RA_ON) == (1))) && (((Mode) == (4))) && (((State) == (0))) && (FRONTEND_CTRL == 1)]
  (junction 1073748338) -> (junction 1073748346) [order 2]
  (junction 1073748340) -> (junction 1073748342) : {
      | reqtable_postcondition((((PACE_CHARGE_CTRL) == (1))) && (VENT_PACE_CTRL == 0) && (((PACING_REF_PWM ) == (VENT_AMP))) && (((PACE_CHARGE_CTRL) == (1))) && (((PACE_GND_CTRL) == (1))) && (VENT_GND_CTRL == 1) && (((RED_LED) == (0))) && (((GREEN_LED) == (0))) && (((BLUE_LED) == (0))) && (VENT_CMP_REF_PWM == Sample_Amp) && (time-oldTime >= PERIOD-5), 'R:14');
      |
      | }
  (junction 1073748342) -> (junction 1073748344) : {
      | }
  (junction 1073748344) -> (junction 1073748346)
  (junction 1073748346) -> (junction 1073748348)
  (junction 1073748348) -> (junction 1073748350) : {
      | % END_R_100
      | }
  (junction 1073748350) -> (junction 1073748352) : {
      | % START_R_25
      | }
  (junction 1073748352) -> (junction 1073748354) : {
      | }
  (junction 1073748354) -> (junction 1073748356)
  (junction 1073748356) -> (junction 1073748358) [order 1] : [(((RA_ON) == (0))) && (((Mode) == (4))) && (((State) == (1)))]
  (junction 1073748356) -> (junction 1073748364) [order 2]
  (junction 1073748358) -> (junction 1073748360) : {
      | reqtable_postcondition((((PACE_CHARGE_CTRL) == (0))) && (VENT_PACE_CTRL == 1) && (((PACING_REF_PWM ) == (VENT_AMP))) && (((PACE_CHARGE_CTRL) == (0))) && (((PACE_GND_CTRL) == (1))) && (VENT_GND_CTRL == 0) && (((RED_LED) == (0))) && (((GREEN_LED) == (1))) && (((BLUE_LED) == (0))) && (VENT_CMP_REF_PWM == Sample_Amp) && (time-oldTime / (60*1000) >= LOWER_RATE), 'R:15');
      |
      | }
  (junction 1073748360) -> (junction 1073748362) : {
      | }
  (junction 1073748362) -> (junction 1073748364)
  (junction 1073748364) -> (junction 1073748366)
  (junction 1073748366) -> (junction 1073748368) : {
      | % END_R_25
      | }
  (junction 1073748368) -> (junction 1073748370) : {
      | % START_R_103
      | }
  (junction 1073748370) -> (junction 1073748372) : {
      | }
  (junction 1073748372) -> (junction 1073748374)
  (junction 1073748374) -> (junction 1073748376) [order 1] : [(((RA_ON) == (1))) && (((Mode) == (4))) && (((State) == (1)))]
  (junction 1073748374) -> (junction 1073748382) [order 2]
  (junction 1073748376) -> (junction 1073748378) : {
      | reqtable_postcondition((((PACE_CHARGE_CTRL) == (0))) && (VENT_PACE_CTRL == 1) && (((PACING_REF_PWM ) == (VENT_AMP))) && (((PACE_CHARGE_CTRL) == (0))) && (((PACE_GND_CTRL) == (1))) && (VENT_GND_CTRL == 0) && (((RED_LED) == (0))) && (((GREEN_LED) == (1))) && (((BLUE_LED) == (0))) && (VENT_CMP_REF_PWM == Sample_Amp) && (time-oldTime >= PERIOD-5), 'R:16');
      |
      | }
  (junction 1073748378) -> (junction 1073748380) : {
      | }
  (junction 1073748380) -> (junction 1073748382)
  (junction 1073748382) -> (junction 1073748384)
  (junction 1073748384) -> (junction 1073748386) : {
      | % END_R_103
      | }
  data: State input; FRONTEND_CTRL input; Mode input; PACE_CHARGE_CTRL input; ATR_AMP input; ATR_GND_CTRL input; ATR_PACE_CTRL input; BLUE_LED input; GREEN_LED input; PACE_GND_CTRL input; PACING_REF_PWM input; RED_LED input; VENT_GND_CTRL input; VENT_PACE_CTRL input; VENT_AMP input; Sample_Amp input; ATR_CMP_REF_PWM input; RA_ON input; LOWER_RATE input; PERIOD input; VENT_CMP_REF_PWM input; time input double [0..]; oldTime constant double =0

== stateflow chart RequirementTable_testing_RA/Modes/Chart ==
  state Identify_Mode_Path
    entry:
    % MODE = 1 (AOO)
    % MODE = 2 (AAI)
    % MODE = 3 (VOO)
    % MODE = 4 (VVI)
    %
    %pacemaker disconnected
    %stop sensing
    PACE_CHARGE_CTRL = LOW
    VENT_PACE_CTRL = LOW
    ATR_PACE_CTRL = LOW
    PACE_GND_CTRL = LOW
    ATR_GND_CTRL = LOW
    VENT_GND_CTRL = LOW
    Z_ATR_CTRL = LOW
    Z_VENT_CTRL = LOW
    FRONTEND_CTRL = LOW
  state AOO
    entry:
    %Charge primary capcitor C22
    ATR_PACE_CTRL=LOW
    PACING_REF_PWM = 20*ATR_Amp
    PACE_CHARGE_CTRL = HIGH
    %Discharge block capacitor C21
    PACE_GND_CTRL = HIGH
    ATR_GND_CTRL = HIGH
    %use LED  to verify state
  state AOO_ATR_PULSE
    entry:
    %Discharge C22 primary capacitor
    %Charge C21 block capacitor
    PACE_CHARGE_CTRL = LOW
    PACE_GND_CTRL = HIGH
    ATR_PACE_CTRL = HIGH
    ATR_GND_CTRL = LOW
    PACING_REF_PWM = 20*ATR_Amp
    %use LED  to verify state
  state AAI
    entry:
    %sensing ON
    FRONTEND_CTRL = HIGH
    %Charge primary capcitor C22
    ATR_PACE_CTRL=LOW
    PACING_REF_PWM = 20*ATR_Amp
    PACE_CHARGE_CTRL = HIGH
    %Discharge block capacitor C21
    PACE_GND_CTRL = HIGH
    ATR_GND_CTRL = HIGH
    ATR_CMP_REF_PWM = Sample_Amp
    %use LED  to verify state
  state AAI_ATR_PULSE
    entry:
    %sensing OFF
    FRONTEND_CTRL = LOW
    %Discharge C22 primary capacitor
    %Charge C21 block capacitor
    PACE_CHARGE_CTRL = LOW
    PACE_GND_CTRL = HIGH
    ATR_PACE_CTRL = HIGH
    ATR_GND_CTRL = LOW
    PACING_REF_PWM = 20*ATR_Amp
    %use LED  to verify state
  state VOO
    entry:
    %Charge primary capcitor C22
    VENT_PACE_CTRL=LOW
    PACING_REF_PWM = 20*VENT_Amp
    PACE_CHARGE_CTRL = HIGH
    %Discharge block capacitor C21
    PACE_GND_CTRL = HIGH
    VENT_GND_CTRL = HIGH
    %use LED  to verify state
  state VOO_VENT_PULSE
    entry:
    %Discharge C22 primary capacitor
    %Charge C21 block capacitor
    PACE_CHARGE_CTRL = LOW
    PACE_GND_CTRL = HIGH
    VENT_GND_CTRL = LOW
    VENT_PACE_CTRL  = HIGH
    PACING_REF_PWM = 20*VENT_Amp
    %use LED  to verify state
  state VVI
    entry:
    %sensing ON
    FRONTEND_CTRL = HIGH
    %Charge primary capcitor C22
    VENT_PACE_CTRL= LOW
    PACING_REF_PWM = 20*VENT_Amp
    PACE_CHARGE_CTRL = HIGH
    %Discharge block capacitor C21
    PACE_GND_CTRL = HIGH
    VENT_PACE_CTRL = LOW
    VENT_GND_CTRL = HIGH
    VENT_CMP_REF_PWM = Sample_Amp
    %use LED  to verify state
  state VVI_VENT_PULSE
    %sensing OFF
    FRONTEND_CTRL = LOW
    %Discharge C22 primary capacitor
    %Charge C21 block capacitor
    PACE_CHARGE_CTRL = LOW
    PACE_GND_CTRL = HIGH
    VENT_GND_CTRL = LOW
    VENT_PACE_CTRL  = HIGH
    PACING_REF_PWM = 20*VENT_Amp
    %use LED  to verify state
  (default) -> Identify_Mode_Path
  AOO -> AOO_ATR_PULSE [order 1] : after(PERIOD - ATR_PULSE_WIDTH,msec)
  Identify_Mode_Path -> AOO [order 1] : [MODE == 1]
  AOO_ATR_PULSE -> AOO : after(ATR_PULSE_WIDTH,msec)
  AOO -> Identify_Mode_Path [order 2] : [MODE ~= 1]
  AAI_ATR_PULSE -> AAI : after(ATR_PULSE_WIDTH,msec)
  Identify_Mode_Path -> AAI [order 2] : [MODE == 2]
  AAI -> (junction 41) [order 1]
  (junction 41) -> AAI_ATR_PULSE [order 1] : after(PERIOD - ATR_PULSE_WIDTH,msec)[ATR_CMP_DETECT == LOW]
  (junction 41) -> AAI [order 2] : after(ATR_RP, msec)[ATR_CMP_DETECT == HIGH]
  AAI -> Identify_Mode_Path [order 2] : [MODE ~= 2]
  VOO -> VOO_VENT_PULSE [order 1] : after(PERIOD - VENT_PULSE_WIDTH,msec)
  Identify_Mode_Path -> VOO [order 3] : [MODE == 3]
  VOO_VENT_PULSE -> VOO : after(VENT_PULSE_WIDTH,msec)
  VOO -> Identify_Mode_Path [order 2] : [MODE ~= 3]
  VVI_VENT_PULSE -> VVI : after(VENT_PULSE_WIDTH,msec)
  Identify_Mode_Path -> VVI [order 4] : [MODE == 4]
  VVI -> (junction 61) [order 1]
  (junction 61) -> VVI_VENT_PULSE [order 1] : after(PERIOD - VENT_PULSE_WIDTH,msec)[VENT_CMP_DETECT == LOW]
  (junction 61) -> VVI [order 2] : after(VENT_RP, msec)[VENT_CMP_DETECT == HIGH]
  VVI -> Identify_Mode_Path [order 2] : [MODE ~= 4]
  data: ATR_PULSE_WIDTH input; PERIOD input; ATR_Amp input; MODE input; VENT_PULSE_WIDTH input; VENT_Amp input; ATR_RP input; Sample_Amp input; VENT_RP input; ATR_CMP_DETECT input; VENT_CMP_DETECT input; HIGH local =1; LOW local =0; ATR_GND_CTRL output; ATR_PACE_CTRL output; PACE_CHARGE_CTRL output; PACE_GND_CTRL output; PACING_REF_PWM output; VENT_GND_CTRL output; VENT_PACE_CTRL output; Z_ATR_CTRL output; Z_VENT_CTRL output; FRONTEND_CTRL output; ATR_CMP_REF_PWM output; VENT_CMP_REF_PWM output
